simulink model "CalculationModel"  (R2013b)
settings: Solver=ode45  StartTime=0.0  StopTime=10.0  RelTol=1e-3
settings Model: Creator=Savnik  LastModifiedBy=Savnik

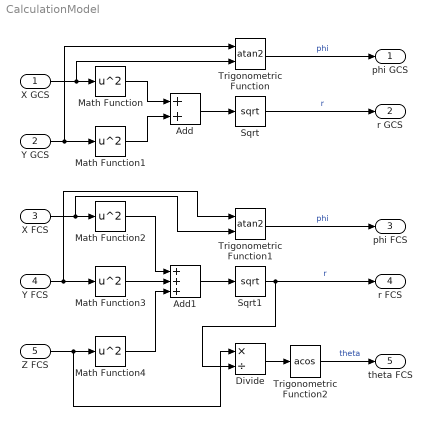
== system CalculationModel ==
  X GCS : Inport
  Y GCS : Inport  Port=2
  X FCS : Inport  Port=3
  Y FCS : Inport  Port=4
  Z FCS : Inport  Port=5
  Add : Sum
  Add1 : Sum  Inputs=+++
  Divide : Product  Inputs=*/
  Math Function{,1..4} (5 alike) : Math  Operator=square  SaturateOnIntegerOverflow=on
  Sqrt : Sqrt  SaturateOnIntegerOverflow=on
  Sqrt1 : Sqrt  SaturateOnIntegerOverflow=on
  Trigonometric Function : Trigonometry  Operator=atan2
  Trigonometric Function1 : Trigonometry  Operator=atan2
  Trigonometric Function2 : Trigonometry  Operator=acos
  phi GCS : Outport
  r GCS : Outport  Port=2
  "phi FCS " : Outport  Port=3
  r FCS : Outport  Port=4
  theta FCS : Outport  Port=5
  wires:
  X GCS/1 -> Trigonometric Function/2, Math Function/1
  Y GCS/1 -> Trigonometric Function/1, Math Function1/1
  Math Function/1 -> Add/1
  Math Function1/1 -> Add/2
  Add/1 -> Sqrt/1
  Math Function2/1 -> Add1/1
  Math Function3/1 -> Add1/2
  Math Function4/1 -> Add1/3
  Add1/1 -> Sqrt1/1
  X FCS/1 -> Trigonometric Function1/2, Math Function2/1
  Y FCS/1 -> Trigonometric Function1/1, Math Function3/1
  Z FCS/1 -> Divide/1, Math Function4/1
  Sqrt/1 -> r GCS/1  "r"
  Sqrt1/1 -> r FCS/1, Divide/2  "r"
  Trigonometric Function/1 -> phi GCS/1  "phi"
  Trigonometric Function1/1 -> "phi FCS "/1  "phi"
  Divide/1 -> Trigonometric Function2/1
  Trigonometric Function2/1 -> theta FCS/1  "theta"
